simulink library "Motor_UL"  (R2019a)
settings: Solver=VariableStepAuto  StartTime=0.0  StopTime=10.0  RelTol=1e-3
undefined symbols (not defined in the file): Motor, VEH
libraries: simulink x2
settings Model: Creator=John Jr  LastModifiedBy=John Jr

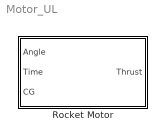
== system Motor_UL ==
  Rocket Motor : Subsystem  mask{F_th=Motor.F_th, t_vec=Motor.T_b, t_b=Motor.t_b, m_m=Motor.m_m, m_f=Motor.m_f, k=Motor.k_m, L=VEH.L1}
      mask prompts: F_th "Thrust curve force vector"; t_vec "Thrust curve time vector"; t_b "Total motor burn time [s]"; m_m "Empty motor mass [kg]"; m_f "Propellant mass [kg]"; k "Motor variance"; L "Vehicle length [m]"
      mask DialogControl DescGroupVar Prompt: Rocket Motor Library
      mask DialogControl DescTextVar Prompt: This block models the motor's thrust acting on the vehicle, including rotational effects.
      mask Display:
      | patch([0 1 1 0], [0 0 1 1],[.8 1 1])
      | 
      | port_label('input',1,'\fontname{Cambria Math}Angle [rad]','texmode','on')
      | port_label('input',2,'\fontname{Cambria Math}Time [s]','texmode','on')
      | port_label('input',3,'\fontname{Cambria Math}CG [m]','texmode','on')
      | 
      | port_label('output',1,'\fontname{Cambria Math}Motor_{out}','texmode','on')

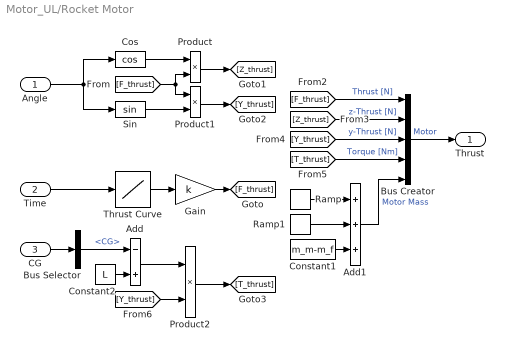
== system Motor_UL/Rocket Motor ==
  Angle : Inport
  Time : Inport  Port=2
  CG : Inport  Port=3
  Add : Sum  Inputs=-+
  Add1 : Sum  Inputs=+++
  Bus Creator : BusCreator  Inputs=5
  Bus Selector : BusSelector  OutputSignals=CG
  Constant1 : Constant  Value=m_m-m_f
  Constant2 : Constant  Value=L
  Cos : Trigonometry  Operator=cos
  Gain : Gain  Gain=k
  Product : Product
  Product1 : Product
  Product2 : Product
  Ramp : simulink/Sources/Ramp  slope=-m_f/t_b  start=0  InitialOutput=m_f
  Ramp1 : simulink/Sources/Ramp  slope=m_f/t_b  start=t_b  InitialOutput=0
  Sin : Trigonometry
  Thrust Curve : Lookup_n-D  NumberOfTableDimensions=1  BreakpointsForDimension1=t_vec  Table=F_th  InternalRulePriority=Speed  RndMeth=Simplest  InputSameDT=on
  Thrust : Outport
  wires:
  Product2/1 -> [T_thrust]
  [Y_thrust] -> Product2/2
  Add/1 -> Product2/1
  Bus Selector/1 -> Add/1  "<CG>"
  Constant2/1 -> Add/2
  CG/1 -> Bus Selector/1
  Thrust Curve/1 -> Gain/1
  Time/1 -> Thrust Curve/1
  Gain/1 -> [F_thrust]
  Angle/1 -> Sin/1, Cos/1
  Cos/1 -> Product/1
  [F_thrust] -> Product1/1, Product/2
  Sin/1 -> Product1/2
  Product/1 -> [Z_thrust]
  Product1/1 -> [Y_thrust]
  Bus Creator/1 -> Thrust/1  "Motor"
  [F_thrust] -> Bus Creator/1  "Thrust [N]"
  [Z_thrust] -> Bus Creator/2  "z-Thrust [N]"
  [Y_thrust] -> Bus Creator/3  "y-Thrust [N]"
  [T_thrust] -> Bus Creator/4  "Torque [Nm]"
  Ramp/1 -> Add1/1
  Constant1/1 -> Add1/3
  Ramp1/1 -> Add1/2
  Add1/1 -> Bus Creator/5  "Motor Mass"
